simulink model "lateral_autopilot_3e"  (R2016b)
settings: Solver=VariableStepAuto  StartTime=0.0  StopTime=t_end  RelTol=1e-3
values from neighbouring files (symbols this model uses):
  A = [ -0.322 0.052 0.028 -1.12 ... (first row only)    [parameters_P3.m]    (also in parameters_longitudal_autopilot.m = [ -0.322 0.052 0.028 -1.12 0.002)
  B = [ 0.002 0 -0.65 -0.02]'    [parameters_P3.m]    (also in parameters_longitudal_autopilot.m = [ 0 0 0 0 10]')
  C = [0 0 1 0 ... (first row only)    [parameters_P3.m]    (also in parameters_longitudal_autopilot.m = [0 0 0 1 0)
  D = [0 0 0]'    [parameters_P3.m]    (also in parameters_longitudal_autopilot.m = [0 0 0 0]')
  d = 2*deg2rad    [run_task_2e.m]    (also in run_task_2f.m; run_task_2g.m = 30*deg2rad)
  delta_a_max = 25*deg2rad    (= 0.436332312999)    [parameters_P3.m]    (also in parameters_longitudal_autopilot.m)
  g = 9.81    [parameters_P3.m]    (also in parameters_longitudal_autopilot.m)
  h = 0.01    [parameters_P3.m]
  integrator_max = 25*deg2rad    (= 0.436332312999)    [parameters_P3.m]    (also in parameters_longitudal_autopilot.m)
  k_d_phi = (2*zeta_phi*omega_n_phi - a_phi_1) / a_phi_2    [parameters_P3.m]    (also in parameters_longitudal_autopilot.m)
  k_i_chi = omega_n_chi^2*V_g/g    [parameters_P3.m]    (also in parameters_longitudal_autopilot.m; regulation_parameters_2_2.m)
  k_i_phi = 0    [parameters_P3.m]    (also in parameters_longitudal_autopilot.m)
  k_p_chi = 2*zeta_chi*omega_n_chi*V_g/g    [parameters_P3.m]    (also in parameters_longitudal_autopilot.m; regulation_parameters_2_2.m)
  k_p_phi = sign(a_phi_2)*delta_a_max /e_phi_max    [parameters_P3.m]    (also in parameters_longitudal_autopilot.m)
  V_g = 637/3.6    (= 176.944444444)    [parameters_P3.m]    (also in parameters_longitudal_autopilot.m)
settings Model: Creator=EllaLovise  LastModifiedBy=EllaLovise

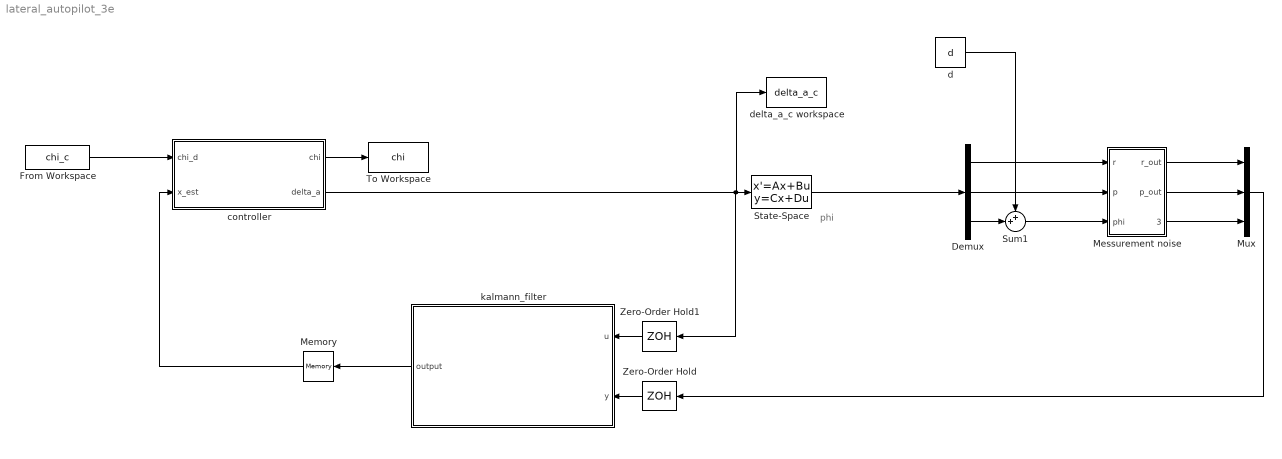
== system lateral_autopilot_3e ==
  note: phi
  Demux : Demux  Outputs=3
  From Workspace : FromWorkspace  VariableName=chi_c  OutputAfterFinalValue=Holding final value
  Memory : Memory
  Messurement noise : Subsystem
  Mux : Mux  Inputs=3
  State-Space : StateSpace  A=A  B=B  C=C  D=D  X0=0
  Sum1 : Sum  Inputs=++|
  To Workspace : ToWorkspace  VariableName=chi  SaveFormat=Structure With Time  SampleTime=-1
  Zero-Order Hold : ZeroOrderHold  SampleTime=h
  Zero-Order Hold1 : ZeroOrderHold  SampleTime=h
  controller : Subsystem
  d : Constant  Value=d
  delta_a_c workspace : ToWorkspace  VariableName=delta_a_c  SaveFormat=Structure With Time  SampleTime=-1
  kalmann_filter : MATLAB Function  TreatAsAtomicUnit=on
  wires:
  State-Space/1 -> Demux/1
  controller/1(chi) -> To Workspace/1
  From Workspace/1 -> controller/1(chi_d)
  Zero-Order Hold/1 -> kalmann_filter/2(y)
  Zero-Order Hold1/1 -> kalmann_filter/1(u)
  controller/2(delta_a) -> delta_a_c workspace/1, State-Space/1, Zero-Order Hold1/1
  kalmann_filter/1(output) -> Memory/1
  Memory/1 -> controller/2(x_est)
  Demux/3 -> Sum1/2
  Demux/1 -> Messurement noise/1(r)
  Demux/2 -> Messurement noise/2(p)
  Sum1/1 -> Messurement noise/3(phi)
  Messurement noise/1(r_out) -> Mux/1
  Messurement noise/2(p_out) -> Mux/2
  Messurement noise/3(phi_out) -> Mux/3
  Mux/1 -> Zero-Order Hold/1
  d/1 -> Sum1/1

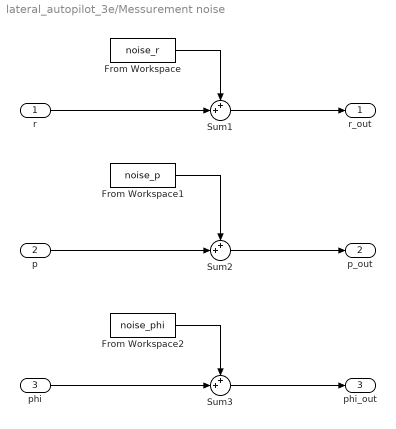
== system lateral_autopilot_3e/Messurement noise ==
  r : Inport
  p : Inport  Port=2
  phi : Inport  Port=3
  From Workspace : FromWorkspace  VariableName=noise_r  OutputAfterFinalValue=Holding final value
  From Workspace1 : FromWorkspace  VariableName=noise_p  OutputAfterFinalValue=Holding final value
  From Workspace2 : FromWorkspace  VariableName=noise_phi  OutputAfterFinalValue=Holding final value
  Sum1 : Sum  Inputs=++|
  Sum2 : Sum  Inputs=++|
  Sum3 : Sum  Inputs=++|
  r_out : Outport
  p_out : Outport  Port=2
  phi_out : Outport  Port=3
  wires:
  p/1 -> Sum2/2
  Sum1/1 -> r_out/1
  Sum2/1 -> p_out/1
  Sum3/1 -> phi_out/1
  From Workspace/1 -> Sum1/1
  r/1 -> Sum1/2
  From Workspace2/1 -> Sum3/1
  From Workspace1/1 -> Sum2/1
  phi/1 -> Sum3/2

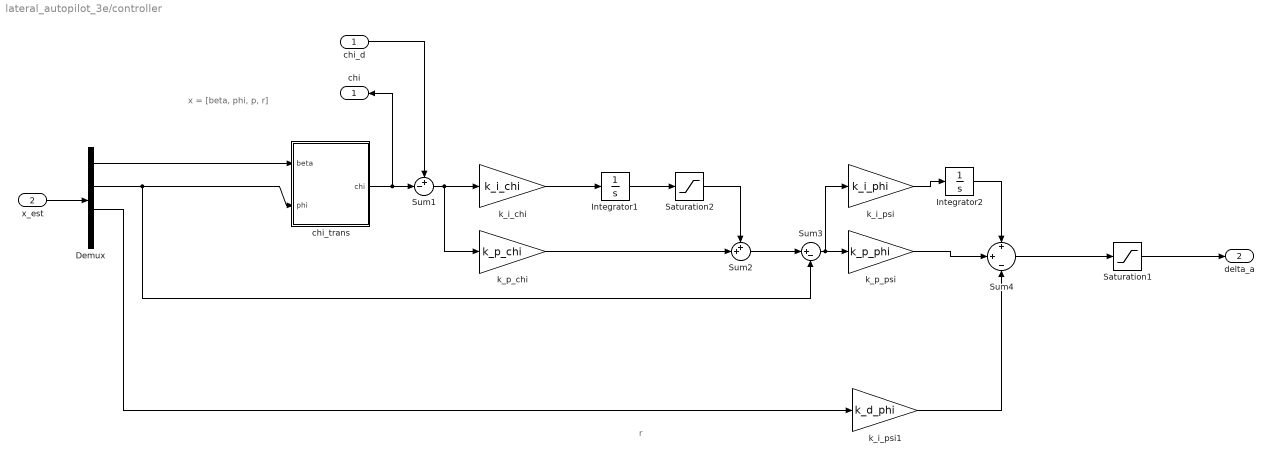
== system lateral_autopilot_3e/controller ==
  note: r
  note: x = [beta, phi, p, r]
  chi_d : Inport
  x_est : Inport  Port=2
  Demux : Demux
  Integrator1 : Integrator
  Integrator2 : Integrator
  Saturation1 : Saturate  UpperLimit=delta_a_max  LowerLimit=-1*delta_a_max
  Saturation2 : Saturate  UpperLimit=integrator_max  LowerLimit=-integrator_max
  Sum1 : Sum  Inputs=+-|
  Sum2 : Sum  Inputs=++|
  Sum3 : Sum  Inputs=|+-
  Sum4 : Sum  Inputs=+|+|-
  chi_trans : Subsystem
  k_i_chi : Gain  Gain=k_i_chi
  k_i_psi : Gain  Gain=k_i_phi
  k_i_psi1 : Gain  Gain=k_d_phi
  k_p_chi : Gain  Gain=k_p_chi
  k_p_psi : Gain  Gain=k_p_phi
  chi : Outport
  delta_a : Outport  Port=2
  wires:
  Demux/2 -> Sum3/2, chi_trans/2(phi)
  k_p_chi/1 -> Sum2/2
  Sum2/1 -> Sum3/1
  Sum3/1 -> k_p_psi/1, k_i_psi/1
  Integrator2/1 -> Sum4/1
  k_i_psi1/1 -> Sum4/3
  k_p_psi/1 -> Sum4/2
  k_i_psi/1 -> Integrator2/1
  Demux/3 -> k_i_psi1/1
  k_i_chi/1 -> Integrator1/1
  Saturation2/1 -> Sum2/1
  Integrator1/1 -> Saturation2/1
  x_est/1 -> Demux/1
  Demux/1 -> chi_trans/1(beta)
  Sum1/1 -> k_p_chi/1, k_i_chi/1
  chi_trans/1(chi) -> chi/1, Sum1/2
  chi_d/1 -> Sum1/1
  Sum4/1 -> Saturation1/1
  Saturation1/1 -> delta_a/1

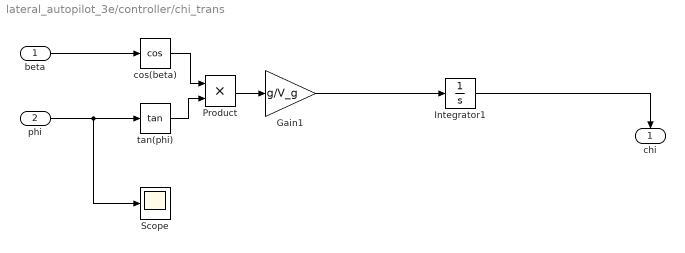
== system lateral_autopilot_3e/controller/chi_trans ==
  beta : Inport
  phi : Inport  Port=2
  Gain1 : Gain  Gain=g/V_g
  Integrator1 : Integrator
  Product : Product
  Scope : Scope
  cos(beta) : Trigonometry  Operator=cos
  tan(phi) : Trigonometry  Operator=tan
  chi : Outport
  wires:
  phi/1 -> Scope/1, tan(phi)/1
  Integrator1/1 -> chi/1
  beta/1 -> cos(beta)/1
  tan(phi)/1 -> Product/2
  Product/1 -> Gain1/1
  cos(beta)/1 -> Product/1
  Gain1/1 -> Integrator1/1

== matlab function lateral_autopilot_3e/kalmann_filter ==
  data: u input; y input; output output; system_information_struct parameter
function output = fcn(u,y, system_information_struct)
persistent P_priori init_flag x_priori

A_d = system_information_struct.A_d;
B_d = system_information_struct.B_d;
E_d = system_information_struct.E_d;
C = system_information_struct.C;
Q = system_information_struct.Q;
I = system_information_struct.I;
R = system_information_struct.R;

if isempty(init_flag) %check if first round 
    init_flag = 1;
    
    P_0_priori= eye(4); 
    x_0_priori = [0; 0; 0; 0];
    P_priori = P_0_priori;
    x_priori = x_0_priori;
end

% 1) Compute Kalman gain
L = P_priori * C' * inv( C * P_priori * C' + R); 

% 2) update error covariance matrix
P = ( I - L*C)*P_priori*( I- L*C)' + L* R*L';

% 3) Update estimate with measurement
x_posteriori = x_priori + L * ( y - C*x_priori);

% 4) Project ahead
x_next_priori = A_d * x_posteriori + B_d*u;
P_next_priori = A_d*P*A_d' + E_d*Q*E_d';

x_priori = x_next_priori;
P_priori = P_next_priori; 

output = x_posteriori;
